simulink model "testersensorow"  (R2022b)
settings: Solver=VariableStepAuto  StartTime=0.0  StopTime=10  RelTol=1e-3
values from neighbouring files (symbols this model uses):
  Np = linspace(0.5,2,101)    [dane.m]    (also in tester23.m; untitled.m = 2303; wykresownik33.m; wykresownik35.m)
  Q = 1./Np    [dane.m]    (also in tester23.m; wykresownik33.m; wykresownik35.m; wykresownik36.m)
settings Model: Creator=48519  LastModifiedBy=48519
settings ModelReferenceCC: EnableRefExpFcnMdlSchedulingChecks=on

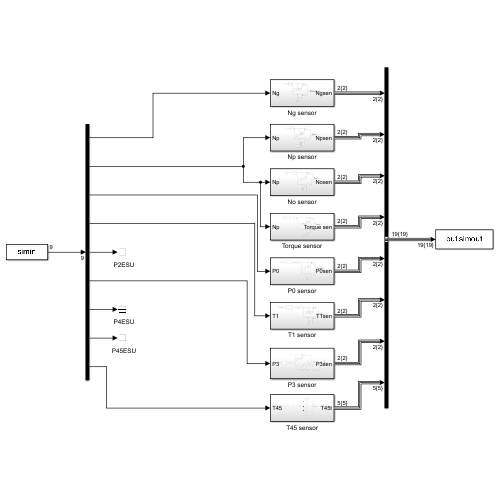
[thumbnail: Simulink's stored preview of the top-level diagram]
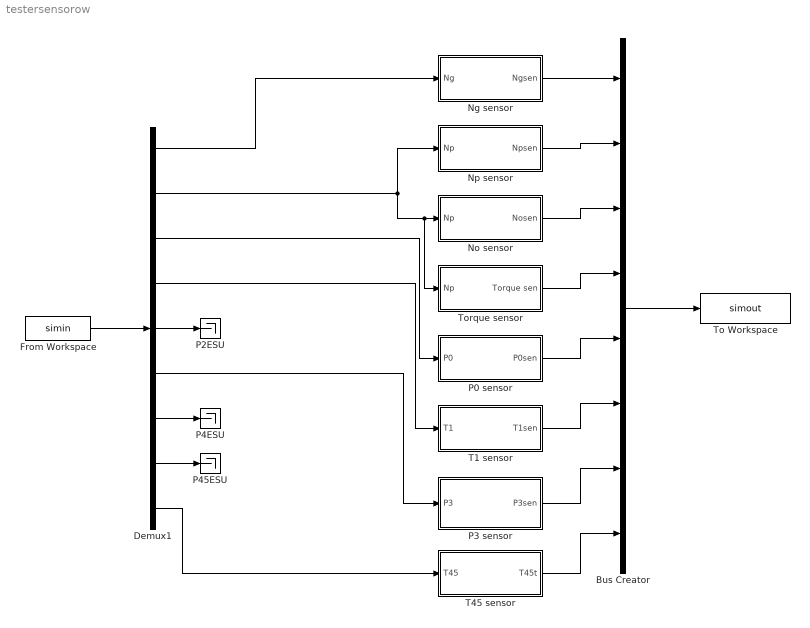
== system testersensorow ==
  Bus Creator : BusCreator  Inputs=8
  Demux1 : Demux  Outputs=9
  From Workspace : FromWorkspace  VariableName=simin
  Ng sensor : Subsystem
  No sensor : Subsystem
  Np sensor : Subsystem
  P0 sensor : Subsystem
  P2ESU : Terminator
  P3 sensor : Subsystem
  P45ESU : Terminator
  P4ESU : Terminator
  T1 sensor : Subsystem
  T45 sensor : Subsystem
  To Workspace : ToWorkspace  VariableName=simout  SaveFormat=Timeseries  SampleTime=-1
  Torque sensor : Subsystem
  wires:
  Demux1/2 -> Np sensor/1(Np), Torque sensor/1(Np), No sensor/1(Np)
  Demux1/1 -> Ng sensor/1(Ng)
  From Workspace/1 -> Demux1/1
  Demux1/8 -> P45ESU/1
  Demux1/3 -> P0 sensor/1(P0)
  Demux1/6 -> P3 sensor/1(P3)
  Demux1/7 -> P4ESU/1
  Demux1/4 -> T1 sensor/1(T1)
  Demux1/5 -> P2ESU/1
  Demux1/9 -> T45 sensor/1(T45)
  Ng sensor/1(Ngsen) -> Bus Creator/1
  No sensor/1(Nosen) -> Bus Creator/3
  Np sensor/1(Npsen) -> Bus Creator/2
  Torque sensor/1(Torque sen) -> Bus Creator/4
  P0 sensor/1(P0sen) -> Bus Creator/5
  T1 sensor/1(T1sen) -> Bus Creator/6
  P3 sensor/1(P3sen) -> Bus Creator/7
  T45 sensor/1(T45t) -> Bus Creator/8
  Bus Creator/1 -> To Workspace/1

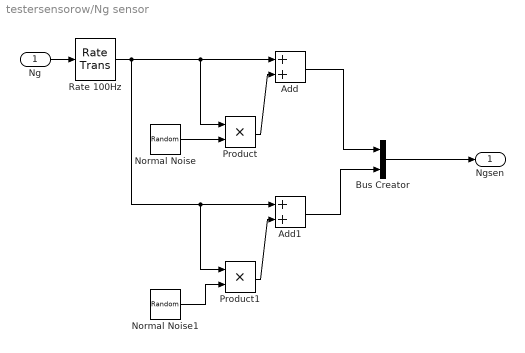
== system testersensorow/Ng sensor ==
  Ng : Inport
  Add : Sum
  Add1 : Sum
  Bus Creator : BusCreator  Inputs=2
  Normal Noise : RandomNumber  Variance=((0.017)^2)*pi/2  Seed=10  SampleTime=0.01
  Normal Noise1 : RandomNumber  Variance=((0.017)^2)*pi/2  Seed=11  SampleTime=0.01
  Product : Product
  Product1 : Product
  Rate 100Hz : RateTransition  OutPortSampleTimeMultiple=2  OutPortSampleTime=0.01
  Ngsen : Outport
  wires:
  Product/1 -> Add/2
  Product1/1 -> Add1/2
  Normal Noise1/1 -> Product1/2
  Rate 100Hz/1 -> Add/1, Product/1, Add1/1, Product1/1
  Ng/1 -> Rate 100Hz/1
  Add1/1 -> Bus Creator/2
  Add/1 -> Bus Creator/1
  Bus Creator/1 -> Ngsen/1
  Normal Noise/1 -> Product/2

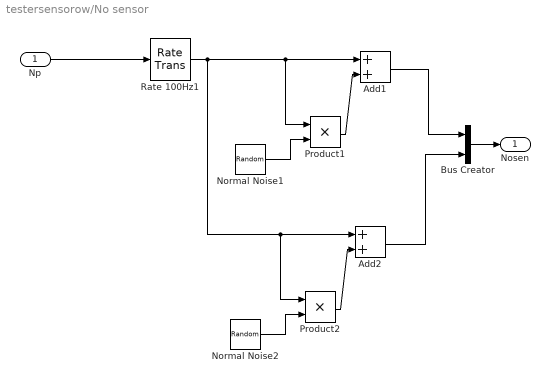
== system testersensorow/No sensor ==
  Np : Inport
  Add1 : Sum
  Add2 : Sum
  Bus Creator : BusCreator  Inputs=2
  Normal Noise1 : RandomNumber  Variance=((0.017)^2)*pi/2  Seed=16  SampleTime=0.01
  Normal Noise2 : RandomNumber  Variance=((0.017)^2)*pi/2  Seed=18  SampleTime=0.01
  Product1 : Product
  Product2 : Product
  Rate 100Hz1 : RateTransition  OutPortSampleTimeMultiple=2  OutPortSampleTime=0.01
  Nosen : Outport
  wires:
  Np/1 -> Rate 100Hz1/1
  Normal Noise2/1 -> Product2/2
  Rate 100Hz1/1 -> Add2/1, Product2/1, Add1/1, Product1/1
  Add2/1 -> Bus Creator/2
  Add1/1 -> Bus Creator/1
  Bus Creator/1 -> Nosen/1
  Normal Noise1/1 -> Product1/2
  Product1/1 -> Add1/2
  Product2/1 -> Add2/2

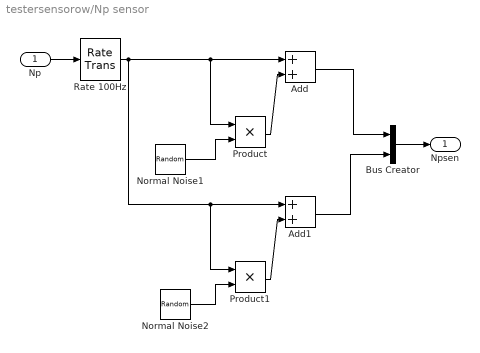
== system testersensorow/Np sensor ==
  Np : Inport
  Add : Sum
  Add1 : Sum
  Bus Creator : BusCreator  Inputs=2
  Normal Noise1 : RandomNumber  Variance=((0.017)^2)*pi/2  Seed=13  SampleTime=0.01
  Normal Noise2 : RandomNumber  Variance=((0.017)^2)*pi/2  Seed=14  SampleTime=0.01
  Product : Product
  Product1 : Product
  Rate 100Hz : RateTransition  OutPortSampleTimeMultiple=2  OutPortSampleTime=0.01
  Npsen : Outport
  wires:
  Normal Noise1/1 -> Product/2
  Product/1 -> Add/2
  Np/1 -> Rate 100Hz/1
  Normal Noise2/1 -> Product1/2
  Product1/1 -> Add1/2
  Rate 100Hz/1 -> Add/1, Product/1, Add1/1, Product1/1
  Add1/1 -> Bus Creator/2
  Add/1 -> Bus Creator/1
  Bus Creator/1 -> Npsen/1

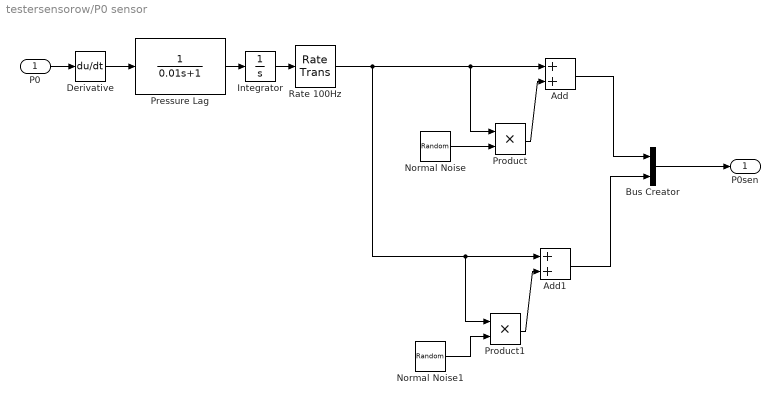
== system testersensorow/P0 sensor ==
  P0 : Inport
  Add : Sum
  Add1 : Sum
  Bus Creator : BusCreator  Inputs=2
  Derivative : Derivative
  Integrator : Integrator  InitialCondition=1
  Normal Noise : RandomNumber  Variance=((0.005)^2)*pi/2  Seed=31  SampleTime=0.01
  Normal Noise1 : RandomNumber  Variance=((0.005)^2)*pi/2  Seed=33  SampleTime=0.01
  Pressure Lag : TransferFcn  Denominator=[0.01 1]
  Product : Product
  Product1 : Product
  Rate 100Hz : RateTransition  OutPortSampleTimeMultiple=2  OutPortSampleTime=0.01
  P0sen : Outport
  wires:
  P0/1 -> Derivative/1
  Normal Noise1/1 -> Product1/2
  Normal Noise/1 -> Product/2
  Add1/1 -> Bus Creator/2
  Pressure Lag/1 -> Integrator/1
  Bus Creator/1 -> P0sen/1
  Product1/1 -> Add1/2
  Product/1 -> Add/2
  Rate 100Hz/1 -> Add1/1, Product1/1, Add/1, Product/1
  Add/1 -> Bus Creator/1
  Derivative/1 -> Pressure Lag/1
  Integrator/1 -> Rate 100Hz/1

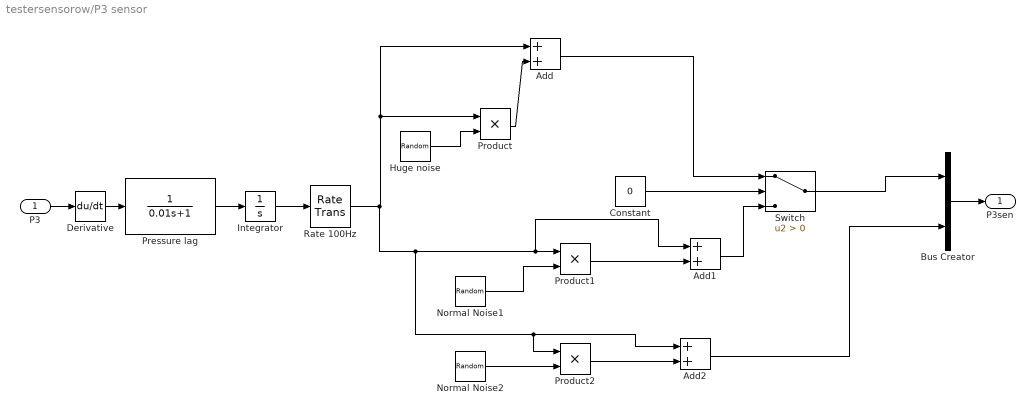
== system testersensorow/P3 sensor ==
  P3 : Inport
  Add : Sum
  Add1 : Sum
  Add2 : Sum
  Bus Creator : BusCreator  Inputs=2
  Constant : Constant  Value=0
  Derivative : Derivative
  Huge noise : RandomNumber  Variance=((0.03)^2)*pi/2  Seed=1  SampleTime=0.01
  Integrator : Integrator  InitialCondition=1
  Normal Noise1 : RandomNumber  Variance=((0.005)^2)*pi/2  Seed=2  SampleTime=0.01
  Normal Noise2 : RandomNumber  Variance=((0.005)^2)*pi/2  Seed=4  SampleTime=0.01
  Pressure lag : TransferFcn  Numerator=[1 ]  Denominator=[0.01 1]
  Product : Product
  Product1 : Product
  Product2 : Product
  Rate 100Hz : RateTransition  OutPortSampleTimeMultiple=2  OutPortSampleTime=0.01
  Switch : Switch  Criteria=u2 > Threshold  SaturateOnIntegerOverflow=off  InputSameDT=off
  P3sen : Outport
  wires:
  Bus Creator/1 -> P3sen/1
  P3/1 -> Derivative/1
  Normal Noise2/1 -> Product2/2
  Add/1 -> Switch/1
  Huge noise/1 -> Product/2
  Add1/1 -> Switch/3
  Product/1 -> Add/2
  Product2/1 -> Add2/2
  Rate 100Hz/1 -> Add2/1, Product2/1, Add1/1, Product1/1, Product/1, Add/1
  Add2/1 -> Bus Creator/2
  Normal Noise1/1 -> Product1/2
  Switch/1 -> Bus Creator/1
  Pressure lag/1 -> Integrator/1
  Constant/1 -> Switch/2
  Product1/1 -> Add1/2
  Derivative/1 -> Pressure lag/1
  Integrator/1 -> Rate 100Hz/1

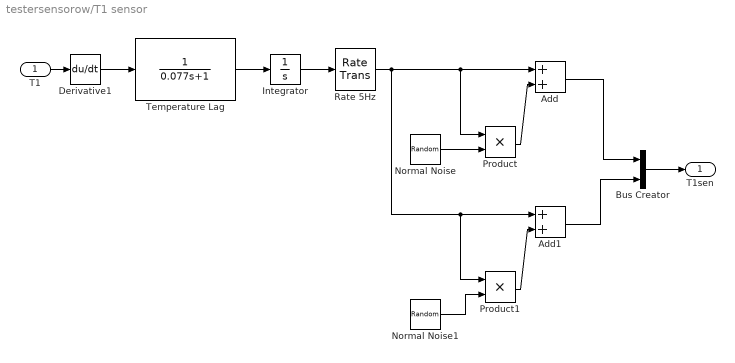
== system testersensorow/T1 sensor ==
  T1 : Inport
  Add : Sum
  Add1 : Sum
  Bus Creator : BusCreator  Inputs=2
  Derivative1 : Derivative
  Integrator : Integrator  InitialCondition=1
  Normal Noise : RandomNumber  Variance=((0.01)^2)*pi/2  Seed=69  SampleTime=0.2
  Normal Noise1 : RandomNumber  Variance=((0.01)^2)*pi/2  Seed=67  SampleTime=0.2
  Product : Product
  Product1 : Product
  Rate 5Hz : RateTransition  OutPortSampleTimeMultiple=2  OutPortSampleTime=0.2
  Temperature Lag : TransferFcn  Denominator=[0.077 1]
  T1sen : Outport
  wires:
  T1/1 -> Derivative1/1
  Temperature Lag/1 -> Integrator/1
  Derivative1/1 -> Temperature Lag/1
  Normal Noise1/1 -> Product1/2
  Normal Noise/1 -> Product/2
  Add1/1 -> Bus Creator/2
  Bus Creator/1 -> T1sen/1
  Rate 5Hz/1 -> Add/1, Product/1, Add1/1, Product1/1
  Add/1 -> Bus Creator/1
  Product1/1 -> Add1/2
  Product/1 -> Add/2
  Integrator/1 -> Rate 5Hz/1

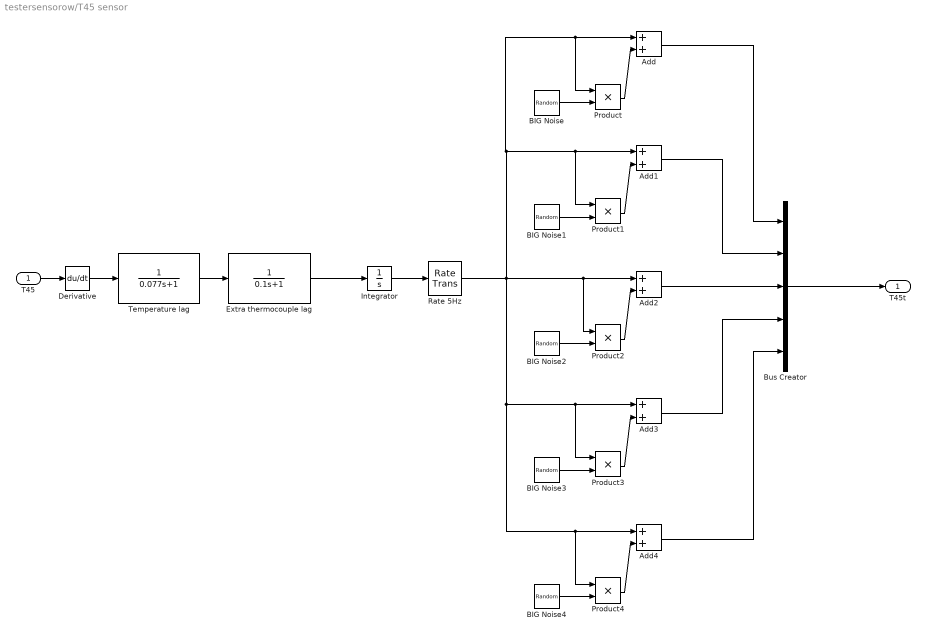
== system testersensorow/T45 sensor ==
  T45 : Inport
  Add{,1..4} (5 alike) : Sum
  BIG Noise : RandomNumber  Variance=((0.015)^2)*pi/2  Seed=51  SampleTime=0.2
  BIG Noise1 : RandomNumber  Variance=((0.015)^2)*pi/2  Seed=53  SampleTime=0.2
  BIG Noise2 : RandomNumber  Variance=((0.015)^2)*pi/2  Seed=55  SampleTime=0.2
  BIG Noise3 : RandomNumber  Variance=((0.015)^2)*pi/2  Seed=57  SampleTime=0.2
  BIG Noise4 : RandomNumber  Variance=((0.015)^2)*pi/2  Seed=59  SampleTime=0.2
  Bus Creator : BusCreator  Inputs=5
  Derivative : Derivative
  Extra thermocouple lag : TransferFcn  Denominator=[0.1 1]
  Integrator : Integrator  InitialCondition=1
  Product{,1..4} (5 alike) : Product
  Rate 5Hz : RateTransition  OutPortSampleTime=0.2
  Temperature lag : TransferFcn  Denominator=[0.077 1]
  T45t : Outport
  wires:
  T45/1 -> Derivative/1
  Extra thermocouple lag/1 -> Integrator/1
  Temperature lag/1 -> Extra thermocouple lag/1
  BIG Noise/1 -> Product/2
  Product/1 -> Add/2
  Product1/1 -> Add1/2
  BIG Noise1/1 -> Product1/2
  Product2/1 -> Add2/2
  BIG Noise2/1 -> Product2/2
  Product3/1 -> Add3/2
  BIG Noise3/1 -> Product3/2
  Product4/1 -> Add4/2
  Rate 5Hz/1 -> Add/1, Product/1, Add1/1, Product1/1, Product2/1, Add2/1, Add3/1, Product3/1, Add4/1, Product4/1
  BIG Noise4/1 -> Product4/2
  Bus Creator/1 -> T45t/1
  Add2/1 -> Bus Creator/3
  Add3/1 -> Bus Creator/4
  Add4/1 -> Bus Creator/5
  Add1/1 -> Bus Creator/2
  Add/1 -> Bus Creator/1
  Integrator/1 -> Rate 5Hz/1
  Derivative/1 -> Temperature lag/1

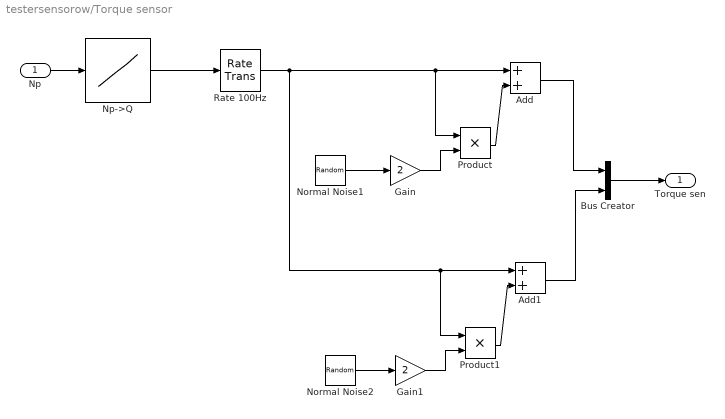
== system testersensorow/Torque sensor ==
  Np : Inport
  Add : Sum
  Add1 : Sum
  Bus Creator : BusCreator  Inputs=2
  Gain : Gain  Gain=2
  Gain1 : Gain  Gain=2
  Normal Noise1 : RandomNumber  Variance=((0.017)^2)*pi/2  Seed=21  SampleTime=0.01
  Normal Noise2 : RandomNumber  Variance=((0.017)^2)*pi/2  Seed=23  SampleTime=0.01
  Np->Q : Lookup_n-D  NumberOfTableDimensions=1  BreakpointsForDimension1=Np  Table=Q  InternalRulePriority=Speed  RndMeth=Simplest
  Product : Product
  Product1 : Product
  Rate 100Hz : RateTransition  OutPortSampleTimeMultiple=2  OutPortSampleTime=0.01
  Torque sen : Outport
  wires:
  Normal Noise1/1 -> Gain/1
  Product/1 -> Add/2
  Gain/1 -> Product/2
  Normal Noise2/1 -> Gain1/1
  Product1/1 -> Add1/2
  Gain1/1 -> Product1/2
  Rate 100Hz/1 -> Add1/1, Product1/1, Add/1, Product/1
  Add1/1 -> Bus Creator/2
  Np/1 -> Np->Q/1
  Add/1 -> Bus Creator/1
  Bus Creator/1 -> Torque sen/1
  Np->Q/1 -> Rate 100Hz/1
